simulink model "ObjectTrackerHDL_ew"  (R2024b)
settings: Solver=VariableStepAuto  StartTime=0.0  StopTime=0.2  RelTol=1e-3  EnableMultiTasking=on
PreLoadFcn:
  | % Blank input
  | img = zeros(480,640);
  | 
  | % Initialize ROI and its center
  | ROI = [175 270 127 127];
  | center = [ROI(2)+(ROI(4)+1)/2 ROI(1)+(ROI(3)+1)/2];
  | 
  | % Template Size
  | templateSize = 128;
  | tSize = templateSize;
  | 
  | % Learning rate
  | eta = 0.075;
  | 
  | % Number of training images
  | trainCount = 2;
  | 
  | % Gaussian Variance
  | sig = 2;
  | 
  | % Generate a Gaussian centered on the first frame
  | iSize = size(img);
  | [x,y] = ndgrid(1:iSize(1), 1:iSize(2));
  | gauss = exp(-((x-center(1)).^2 + (y-center(2)).^2)./(2*sig));
  | gauss = mat2gray(gauss);
  | 
  | % Generate the first template
  | img = imcrop(img, ROI);
  | gauss = imcrop(gauss, ROI);
  | 
  | % Generate the preprocess windowing function
  | [w1,w2] = meshgrid(window(@hann,tSize),window(@hann,tSize));
  | win = w1.*w2;
  | 
  | % Blank initial coefficients
  | G = zeros(tSize,tSize);
  | Ai = zeros(tSize,tSize);
  | Bi = zeros(tSize,tSize);
  | Hi = zeros(tSize,tSize);
  | 
  | numRows = tSize;
  | numCols = tSize;
InitFcn:
  | % Read the first frame
  | vidFReader = VideoReader(get_param('ObjectTrackerHDL/Input','inputFilename'));
  | img = read(vidFReader,1);
  | if (size(img,3) == 3)
  |     img = rgb2gray(img);
  | end
  | img = double(img);
  | 
  | % Initialize Object Center
  | objectCenter = str2num(get_param('ObjectTrackerHDL/ObjectTrackerHDL','objectCenter'));
  | 
  | % Template Size
  | templateSize = str2num(get_param('ObjectTrackerHDL/ObjectTrackerHDL','templateSize'));
  | originROI = objectCenter-templateSize/2;
  | tSize = templateSize;
  | 
  | % Initialize ROI and its center
  | ROI = [originROI tSize-1 tSize-1];
  | center = [ROI(2)+(ROI(4)+1)/2 ROI(1)+(ROI(3)+1)/2];
  | 
  | % Learning rate
  | eta = 0.075;
  | 
  | % Number of training images
  | trainCount = 128;
  | 
  | % Gaussian Variance
  | sig = 2;
  | 
  | % Generate a Gaussian centered on the first frame
  | iSize = size(img);
  | [x,y] = ndgrid(1:iSize(1), 1:iSize(2));
  | gauss = exp(-((x-center(1)).^2 + (y-center(2)).^2)./(2*sig));
  | gauss = mat2gray(gauss);
  | 
  | % Generate the first template
  | img = imcrop(img, ROI);
  | gauss = imcrop(gauss, ROI);
  | 
  | % Generate the preprocess windowing function
  | [w1,w2] = meshgrid(window(@hann,tSize),window(@hann,tSize));
  | win = w1.*w2;
  | 
  | % Preprocessing the first template
  | hgamma = vision.GammaCorrector(2.0,'Correction','De-gamma');
  | img = hgamma(uint8(img));
  | img = double(img);
  | mean1 = mean(img(:));
  | std1 = std(img(:));
  | img = (img-mean1)/std1;
  | fii = img.*win;
  | 
  | % Convert to frequency domain and calculate initial coefficients
  | G = fft2(gauss);
  | Ai = (G.*conj(fft2(fii)));
  | Bi = real((fft2(fii).*conj(fft2(fii))));
  | 
  | rng('default');
  | % Initial training procedure
  | for i = 1:trainCount
  | ... (+19 lines)
model workspace (MAT data in the model file):
  mwTaskManagerKernelLatency = 0
undefined symbols (not defined in the file): a, b, c, Rec, SDTV
libraries: hdlsllib x61, simulink x17, visionhdlutilities x8, visionstatistics x6, dsphdlxfrm2 x6, visionconversions x4, visiontransforms x3, visionhdlio x2, visionhdlconversions x2, visionhdlstatistics x2, visionanalysis x2, visionsinks x1
(part 3 of 3)

== system ObjectTrackerHDL_ew/ObjectTrackerHDL/Track/2-DCorrelation/Prev2-DFFT/pixelBusGenerator ==
  validIn : Inport
  Horizontal : hdlsllib/Sources/HDL Counter  CountType=Count limited  CountInit=0  CountStep=1  CountMax=hEnd  CountFromType=Initial value  CountFrom=0  CountResetPort=off  CountLoadPort=off  CountEnbPort=on  CountDirPort=off  CountHitOutputPort=off  CountDataType=Unsigned  CountWordLen=ceil(log2(hEnd))  CountFracLen=0  CountSampTime=1
  Logical Operator{3..6} (4 alike) : Logic  AllPortsSameDT=off  OutDataTypeStr=boolean
  Pixel Control Bus Creator : visionhdlutilities/Pixel Control Bus Creator
  Vertical : hdlsllib/Sources/HDL Counter  CountType=Count limited  CountInit=0  CountStep=1  CountMax=vEnd  CountFromType=Initial value  CountFrom=0  CountResetPort=off  CountLoadPort=off  CountEnbPort=on  CountDirPort=off  CountHitOutputPort=off  CountDataType=Unsigned  CountWordLen=ceil(log2(vEnd))  CountFracLen=0  CountSampTime=1
  hEnd : simulink/Logic and Bit Operations/Compare To Constant  relop===  const=hEnd  OutDataTypeStr=boolean
  hStart : simulink/Logic and Bit Operations/Compare To Constant  relop===  const=0  OutDataTypeStr=boolean
  vEnd : simulink/Logic and Bit Operations/Compare To Constant  relop===  const=vEnd  OutDataTypeStr=boolean
  vStart : simulink/Logic and Bit Operations/Compare To Constant  relop===  const=0  OutDataTypeStr=boolean
  busOut : Outport  VectorParamsAs1DForOutWhenUnconnected=off
  frameDone : Outport  Port=2  VectorParamsAs1DForOutWhenUnconnected=off
  wires:
  validIn/1 -> Pixel Control Bus Creator/5, Vertical/1, Logical Operator4/1, Logical Operator5/1, Logical Operator6/1, Logical Operator3/1, Horizontal/1
  Horizontal/1 -> hEnd/1, hStart/1
  hEnd/1 -> Logical Operator4/2
  Vertical/1 -> vStart/1, vEnd/1
  vStart/1 -> Logical Operator5/2
  vEnd/1 -> Logical Operator6/2
  Logical Operator5/1 -> Pixel Control Bus Creator/3
  Logical Operator3/1 -> Pixel Control Bus Creator/1
  Logical Operator4/1 -> Pixel Control Bus Creator/2
  hStart/1 -> Logical Operator3/2
  Logical Operator6/1 -> frameDone/1, Pixel Control Bus Creator/4
  Pixel Control Bus Creator/1 -> busOut/1

== system ObjectTrackerHDL_ew/ObjectTrackerHDL/Track/2-DCorrelation/2-DIFFT/CornerTurnMemory/BankBit ==
  addrIn : Inport
  Bit Slice1 : hdlsllib/Logic and Bit Operations/Bit Slice  lidx=(log2(numCols)+log2(numRows))  ridx=(log2(numCols)+log2(numRows))
  Logical Operator3 : Logic  Operator=NOT  IconShape=distinctive  AllPortsSameDT=off  OutDataTypeStr=boolean
  bankWr : Outport  VectorParamsAs1DForOutWhenUnconnected=off
  wires:
  Logical Operator3/1 -> bankWr/1
  Bit Slice1/1 -> Logical Operator3/1
  addrIn/1 -> Bit Slice1/1

== system ObjectTrackerHDL_ew/ObjectTrackerHDL/Track/2-DCorrelation/2-DIFFT/CornerTurnMemory/LowerRAM ==
  din : Inport
  wr_addr : Inport  Port=2
  wr_en : Inport  Port=3
  rd_addr : Inport  Port=4
  complexDataConcat : MATLABSystem  System=hdl.RAM  RAMType=Simple dual port  AsyncRead=off  WriteOutputValue=New data  RAMInitialValue=0  allowBusInputs=off  WritesHaveOutput=on  NumReads=0  NumWrites=1  SimulateUsing=Code generation  ModelRAMDelay=on
      mask Type: hdl.RAM
      mask Display:
      | disp(['Simple' char(10) 'Dual Port' char(10) 'RAM']);
      | port_label('input',1,'din');
      | port_label('input',2,'wr_addr');
      | port_label('input',3,'we');
      | port_label('input',4,'rd_addr');
      | port_label('output',1,'dout');
  dout : Outport  VectorParamsAs1DForOutWhenUnconnected=off
  wires:
  wr_addr/1 -> complexDataConcat/2
  wr_en/1 -> complexDataConcat/3
  rd_addr/1 -> complexDataConcat/4
  din/1 -> complexDataConcat/1
  complexDataConcat/1 -> dout/1

== system ObjectTrackerHDL_ew/ObjectTrackerHDL/Track/2-DCorrelation/2-DIFFT/CornerTurnMemory/SwapAddr ==
  addrIn : Inport
  Bit Concat : hdlsllib/Logic and Bit Operations/Bit Concat  numInputs=2
  Bit Shift : hdlsllib/Logic and Bit Operations/Bit Shift  mode=Shift Left Logical  N=log2(numCols)
  Bit Slice : hdlsllib/Logic and Bit Operations/Bit Slice  lidx=(log2(numCols)+log2(numRows))-1  ridx=log2(numCols)
  Logical Operator3 : Logic  Operator=NOT  IconShape=distinctive  AllPortsSameDT=off  OutDataTypeStr=boolean
  bankBit : hdlsllib/Logic and Bit Operations/Bit Slice  lidx=(log2(numCols)+log2(numRows))  ridx=(log2(numCols)+log2(numRows))
  upperBits : hdlsllib/Logic and Bit Operations/Bit Slice  lidx=(log2(numCols)+log2(numRows))-1  ridx=log2(numCols)
  bankRd : Outport  VectorParamsAs1DForOutWhenUnconnected=off
  addrRd : Outport  Port=2  VectorParamsAs1DForOutWhenUnconnected=off
  wires:
  Bit Concat/1 -> addrRd/1
  upperBits/1 -> Bit Concat/2
  addrIn/1 -> Bit Shift/1, bankBit/1, upperBits/1
  bankBit/1 -> Logical Operator3/1
  Logical Operator3/1 -> bankRd/1
  Bit Shift/1 -> Bit Slice/1
  Bit Slice/1 -> Bit Concat/1

== system ObjectTrackerHDL_ew/ObjectTrackerHDL/Track/2-DCorrelation/2-DIFFT/CornerTurnMemory/UpperRAM ==
  din : Inport
  wr_addr : Inport  Port=2
  wr_en : Inport  Port=3
  rd_addr : Inport  Port=4
  complexDataConcat : MATLABSystem  System=hdl.RAM  RAMType=Simple dual port  AsyncRead=off  WriteOutputValue=New data  RAMInitialValue=0  allowBusInputs=off  WritesHaveOutput=on  NumReads=0  NumWrites=1  SimulateUsing=Code generation  ModelRAMDelay=on
      mask Type: hdl.RAM
      mask Display:
      | disp(['Simple' char(10) 'Dual Port' char(10) 'RAM']);
      | port_label('input',1,'din');
      | port_label('input',2,'wr_addr');
      | port_label('input',3,'we');
      | port_label('input',4,'rd_addr');
      | port_label('output',1,'dout');
  dout : Outport  VectorParamsAs1DForOutWhenUnconnected=off
  wires:
  complexDataConcat/1 -> dout/1
  din/1 -> complexDataConcat/1
  rd_addr/1 -> complexDataConcat/4
  wr_en/1 -> complexDataConcat/3
  wr_addr/1 -> complexDataConcat/2

== system ObjectTrackerHDL_ew/ObjectTrackerHDL/Track/2-DCorrelation/CoefficientsUpdate/CoefficientsUpdate/ComplexDivide ==
  Dividend : Inport
  Divisor : Inport  Port=2
  Complex to Real-Imag : ComplexToRealImag
  Data Type Conversion : DataTypeConversion  OutDataTypeStr=fixdt(1,44,16)  SaturateOnIntegerOverflow=off  RndMeth=Floor
  Data Type Conversion1 : DataTypeConversion  OutDataTypeStr=fixdt(1,44,16)  SaturateOnIntegerOverflow=off  RndMeth=Floor
  Delay14 : Delay  DelayLength=1+52  InitialCondition=0
  Delay15 : Delay  DelayLength=1+52  InitialCondition=0
  Divide3 : Product  Inputs=*/  OutDataTypeStr=fixdt(1,24,12)  RndMeth=Simplest  SaturateOnIntegerOverflow=on
  Divide4 : Product  Inputs=*/  OutDataTypeStr=fixdt(1,24,12)  RndMeth=Simplest  SaturateOnIntegerOverflow=on
  Real-Imag to Complex : RealImagToComplex
  Quotient : Outport
  wires:
  Divide3/1 -> Delay14/1
  Dividend/1 -> Complex to Real-Imag/1
  Data Type Conversion1/1 -> Divide4/1
  Complex to Real-Imag/2 -> Data Type Conversion1/1
  Delay14/1 -> Real-Imag to Complex/1
  Real-Imag to Complex/1 -> Quotient/1
  Data Type Conversion/1 -> Divide3/1
  Delay15/1 -> Real-Imag to Complex/2
  Divisor/1 -> Divide4/2, Divide3/2
  Divide4/1 -> Delay15/1
  Complex to Real-Imag/1 -> Data Type Conversion/1

== system ObjectTrackerHDL_ew/ObjectTrackerHDL/Track/2-DCorrelation/Curr2-DFFT/CornerTurnMemory/BankBit ==
  addrIn : Inport
  Bit Slice1 : hdlsllib/Logic and Bit Operations/Bit Slice  lidx=(log2(numCols)+log2(numRows))  ridx=(log2(numCols)+log2(numRows))
  Logical Operator3 : Logic  Operator=NOT  IconShape=distinctive  AllPortsSameDT=off  OutDataTypeStr=boolean
  bankWr : Outport  VectorParamsAs1DForOutWhenUnconnected=off
  wires:
  Logical Operator3/1 -> bankWr/1
  Bit Slice1/1 -> Logical Operator3/1
  addrIn/1 -> Bit Slice1/1

== system ObjectTrackerHDL_ew/ObjectTrackerHDL/Track/2-DCorrelation/Curr2-DFFT/CornerTurnMemory/LowerRAM ==
  din : Inport
  wr_addr : Inport  Port=2
  wr_en : Inport  Port=3
  rd_addr : Inport  Port=4
  complexDataConcat : MATLABSystem  System=hdl.RAM  RAMType=Simple dual port  AsyncRead=off  WriteOutputValue=New data  RAMInitialValue=0  allowBusInputs=off  WritesHaveOutput=on  NumReads=0  NumWrites=1  SimulateUsing=Code generation  ModelRAMDelay=on
      mask Type: hdl.RAM
      mask Display:
      | disp(['Simple' char(10) 'Dual Port' char(10) 'RAM']);
      | port_label('input',1,'din');
      | port_label('input',2,'wr_addr');
      | port_label('input',3,'we');
      | port_label('input',4,'rd_addr');
      | port_label('output',1,'dout');
  dout : Outport  VectorParamsAs1DForOutWhenUnconnected=off
  wires:
  wr_addr/1 -> complexDataConcat/2
  wr_en/1 -> complexDataConcat/3
  rd_addr/1 -> complexDataConcat/4
  din/1 -> complexDataConcat/1
  complexDataConcat/1 -> dout/1

== system ObjectTrackerHDL_ew/ObjectTrackerHDL/Track/2-DCorrelation/Curr2-DFFT/CornerTurnMemory/SwapAddr ==
  addrIn : Inport
  Bit Concat : hdlsllib/Logic and Bit Operations/Bit Concat  numInputs=2
  Bit Shift : hdlsllib/Logic and Bit Operations/Bit Shift  mode=Shift Left Logical  N=log2(numCols)
  Bit Slice : hdlsllib/Logic and Bit Operations/Bit Slice  lidx=(log2(numCols)+log2(numRows))-1  ridx=log2(numCols)
  Logical Operator3 : Logic  Operator=NOT  IconShape=distinctive  AllPortsSameDT=off  OutDataTypeStr=boolean
  bankBit : hdlsllib/Logic and Bit Operations/Bit Slice  lidx=(log2(numCols)+log2(numRows))  ridx=(log2(numCols)+log2(numRows))
  upperBits : hdlsllib/Logic and Bit Operations/Bit Slice  lidx=(log2(numCols)+log2(numRows))-1  ridx=log2(numCols)
  bankRd : Outport  VectorParamsAs1DForOutWhenUnconnected=off
  addrRd : Outport  Port=2  VectorParamsAs1DForOutWhenUnconnected=off
  wires:
  Bit Concat/1 -> addrRd/1
  upperBits/1 -> Bit Concat/2
  addrIn/1 -> Bit Shift/1, bankBit/1, upperBits/1
  bankBit/1 -> Logical Operator3/1
  Logical Operator3/1 -> bankRd/1
  Bit Shift/1 -> Bit Slice/1
  Bit Slice/1 -> Bit Concat/1

== system ObjectTrackerHDL_ew/ObjectTrackerHDL/Track/2-DCorrelation/Curr2-DFFT/CornerTurnMemory/UpperRAM ==
  din : Inport
  wr_addr : Inport  Port=2
  wr_en : Inport  Port=3
  rd_addr : Inport  Port=4
  complexDataConcat : MATLABSystem  System=hdl.RAM  RAMType=Simple dual port  AsyncRead=off  WriteOutputValue=New data  RAMInitialValue=0  allowBusInputs=off  WritesHaveOutput=on  NumReads=0  NumWrites=1  SimulateUsing=Code generation  ModelRAMDelay=on
      mask Type: hdl.RAM
      mask Display:
      | disp(['Simple' char(10) 'Dual Port' char(10) 'RAM']);
      | port_label('input',1,'din');
      | port_label('input',2,'wr_addr');
      | port_label('input',3,'we');
      | port_label('input',4,'rd_addr');
      | port_label('output',1,'dout');
  dout : Outport  VectorParamsAs1DForOutWhenUnconnected=off
  wires:
  complexDataConcat/1 -> dout/1
  din/1 -> complexDataConcat/1
  rd_addr/1 -> complexDataConcat/4
  wr_en/1 -> complexDataConcat/3
  wr_addr/1 -> complexDataConcat/2

== system ObjectTrackerHDL_ew/ObjectTrackerHDL/Track/2-DCorrelation/Prev2-DFFT/CornerTurnMemory/BankBit ==
  addrIn : Inport
  Bit Slice1 : hdlsllib/Logic and Bit Operations/Bit Slice  lidx=(log2(numCols)+log2(numRows))  ridx=(log2(numCols)+log2(numRows))
  Logical Operator3 : Logic  Operator=NOT  IconShape=distinctive  AllPortsSameDT=off  OutDataTypeStr=boolean
  bankWr : Outport  VectorParamsAs1DForOutWhenUnconnected=off
  wires:
  Logical Operator3/1 -> bankWr/1
  Bit Slice1/1 -> Logical Operator3/1
  addrIn/1 -> Bit Slice1/1

== system ObjectTrackerHDL_ew/ObjectTrackerHDL/Track/2-DCorrelation/Prev2-DFFT/CornerTurnMemory/LowerRAM ==
  din : Inport
  wr_addr : Inport  Port=2
  wr_en : Inport  Port=3
  rd_addr : Inport  Port=4
  complexDataConcat : MATLABSystem  System=hdl.RAM  RAMType=Simple dual port  AsyncRead=off  WriteOutputValue=New data  RAMInitialValue=0  allowBusInputs=off  WritesHaveOutput=on  NumReads=0  NumWrites=1  SimulateUsing=Code generation  ModelRAMDelay=on
      mask Type: hdl.RAM
      mask Display:
      | disp(['Simple' char(10) 'Dual Port' char(10) 'RAM']);
      | port_label('input',1,'din');
      | port_label('input',2,'wr_addr');
      | port_label('input',3,'we');
      | port_label('input',4,'rd_addr');
      | port_label('output',1,'dout');
  dout : Outport  VectorParamsAs1DForOutWhenUnconnected=off
  wires:
  wr_addr/1 -> complexDataConcat/2
  wr_en/1 -> complexDataConcat/3
  rd_addr/1 -> complexDataConcat/4
  din/1 -> complexDataConcat/1
  complexDataConcat/1 -> dout/1

== system ObjectTrackerHDL_ew/ObjectTrackerHDL/Track/2-DCorrelation/Prev2-DFFT/CornerTurnMemory/SwapAddr ==
  addrIn : Inport
  Bit Concat : hdlsllib/Logic and Bit Operations/Bit Concat  numInputs=2
  Bit Shift : hdlsllib/Logic and Bit Operations/Bit Shift  mode=Shift Left Logical  N=log2(numCols)
  Bit Slice : hdlsllib/Logic and Bit Operations/Bit Slice  lidx=(log2(numCols)+log2(numRows))-1  ridx=log2(numCols)
  Logical Operator3 : Logic  Operator=NOT  IconShape=distinctive  AllPortsSameDT=off  OutDataTypeStr=boolean
  bankBit : hdlsllib/Logic and Bit Operations/Bit Slice  lidx=(log2(numCols)+log2(numRows))  ridx=(log2(numCols)+log2(numRows))
  upperBits : hdlsllib/Logic and Bit Operations/Bit Slice  lidx=(log2(numCols)+log2(numRows))-1  ridx=log2(numCols)
  bankRd : Outport  VectorParamsAs1DForOutWhenUnconnected=off
  addrRd : Outport  Port=2  VectorParamsAs1DForOutWhenUnconnected=off
  wires:
  Bit Concat/1 -> addrRd/1
  upperBits/1 -> Bit Concat/2
  addrIn/1 -> Bit Shift/1, bankBit/1, upperBits/1
  bankBit/1 -> Logical Operator3/1
  Logical Operator3/1 -> bankRd/1
  Bit Shift/1 -> Bit Slice/1
  Bit Slice/1 -> Bit Concat/1

== system ObjectTrackerHDL_ew/ObjectTrackerHDL/Track/2-DCorrelation/Prev2-DFFT/CornerTurnMemory/UpperRAM ==
  din : Inport
  wr_addr : Inport  Port=2
  wr_en : Inport  Port=3
  rd_addr : Inport  Port=4
  complexDataConcat : MATLABSystem  System=hdl.RAM  RAMType=Simple dual port  AsyncRead=off  WriteOutputValue=New data  RAMInitialValue=0  allowBusInputs=off  WritesHaveOutput=on  NumReads=0  NumWrites=1  SimulateUsing=Code generation  ModelRAMDelay=on
      mask Type: hdl.RAM
      mask Display:
      | disp(['Simple' char(10) 'Dual Port' char(10) 'RAM']);
      | port_label('input',1,'din');
      | port_label('input',2,'wr_addr');
      | port_label('input',3,'we');
      | port_label('input',4,'rd_addr');
      | port_label('output',1,'dout');
  dout : Outport  VectorParamsAs1DForOutWhenUnconnected=off
  wires:
  complexDataConcat/1 -> dout/1
  din/1 -> complexDataConcat/1
  rd_addr/1 -> complexDataConcat/4
  wr_en/1 -> complexDataConcat/3
  wr_addr/1 -> complexDataConcat/2

== matlab function ObjectTrackerHDL_ew/ObjectTrackerHDL/Track/2-DCorrelation/Prev2-DFFT/CornerTurnMemory/CounterDelay ==
  settings: fimath=hdlfimath
  data: vld_in input boolean; vld_out output boolean; DELAY parameter; templateSize parameter; blanking parameter
function vld_out = cntr_delay(vld_in, DELAY, templateSize, blanking)

CNTR_NT = numerictype(0,nextpow2(DELAY+2),0);
FCNTR_NT = numerictype(0,nextpow2(DELAY),0);
FM = hdlfimath;

persistent wr_cntr rd_cntr rdrw_cntr rdbl_cntr flush_cntr state

STATE_FILL = coder.const(0);
STATE_FLUSH = coder.const(1);
STATE_RESET = coder.const(3);

if isempty(wr_cntr)
    wr_cntr = fi(0,CNTR_NT, FM);
    rd_cntr = fi(0,CNTR_NT, FM);
    rdrw_cntr = fi(0,CNTR_NT, FM);
    rdbl_cntr = fi(0,CNTR_NT, FM);
    flush_cntr = fi(0,FCNTR_NT,FM);
    state = fi(STATE_FILL, 0, 2, 0);
end

%dcount = fi(wr_cntr-rd_cntr,CNTR_NT, FM);

vld_out = false;

switch state
    case STATE_FILL
        if wr_cntr == DELAY
            vld_out = true;
            state(:) = STATE_FLUSH;
            flush_cntr(:) = DELAY-1;
            rd_cntr(:) = rd_cntr + 1;
            rdrw_cntr(:) = rdrw_cntr + 1;
            wr_cntr(:) = 0;
        else
            vld_out = false;
        end
    case STATE_FLUSH
        if flush_cntr == 1
            state(:) = STATE_RESET;
        end 
        if rdrw_cntr < templateSize
        rd_cntr(:) = rd_cntr + 1;
        rdrw_cntr(:) = rdrw_cntr + 1;
        flush_cntr(:) = flush_cntr -1;
        vld_out = true;
        else
        rdbl_cntr(:) = rdbl_cntr(:) + 1;
        vld_out = false;
        end
        if rdbl_cntr >=(blanking-templateSize)
        rdrw_cntr(:) = 0;
        rdbl_cntr(:) = 0;
        end
    case STATE_RESET
        if wr_cntr == DELAY %* 2 -1 
            state(:) = STATE_FILL;
%          if rd_cntr ~= DELAY
%              disp(rd_cntr);
%             error('Out of sync Counter (RD)');
%          end
         rd_cntr(:) = 0;
%          if wr_cntr ~= DELAY
%              disp(wr_cntr);
%             error('Out of sync Counter (WR)');
%          end
        %wr_cntr(:) = 0;
        flush_cntr(:) = DELAY-1;
        else 
            state(:) = STATE_RESET;
        end
end

if vld_in
    wr_cntr(:) = wr_cntr + 1;
end

== matlab function ObjectTrackerHDL_ew/ObjectTrackerHDL/Overlay/VideoOverlay/MATLAB Function ==
  data: position input; Color output; AddShape output; rowCount input; colCount input; colorValue input; lineWidth input
function [Color, AddShape] = InsertRectangle(position, rowCount, colCount, colorValue, lineWidth)
%#codegen


halfLineWidth = int32(bitshift(lineWidth,-1));

Color = uint8(colorValue);%[255 255 0]
% position must not be a column vector
% [x y width]
objectLocAndWidth = int32(position(:,1:4));
objectLocTopStart = objectLocAndWidth(:,1) - int32(halfLineWidth);
objectLocTopEnd = objectLocAndWidth(:,1) + int32(halfLineWidth);
objectLocBottomStart = objectLocAndWidth(:,1) - int32(halfLineWidth)+ objectLocAndWidth(:,3);
objectLocBottomEnd = objectLocAndWidth(:,1) + int32(halfLineWidth)+ objectLocAndWidth(:,3);
objectLocLeftStart = objectLocAndWidth(:,2) - int32(halfLineWidth);
objectLocLeftEnd = objectLocAndWidth(:,2) + int32(halfLineWidth);
objectLocRightStart = objectLocAndWidth(:,2) - int32(halfLineWidth) + objectLocAndWidth(:,4);
objectLocRightEnd = objectLocAndWidth(:,2) + int32(halfLineWidth) + objectLocAndWidth(:,4);

AddShapeHorLimit = (rowCount>=objectLocTopStart) & (rowCount<=objectLocBottomEnd);
AddShapeVerLimit = (colCount>=objectLocLeftStart) & (colCount<=objectLocRightEnd);

AddShapeHor = ((((rowCount>=objectLocTopStart) & (rowCount<=objectLocTopEnd)) | ((rowCount>=objectLocBottomStart) & (rowCount<=objectLocBottomEnd))) & AddShapeVerLimit);
AddShapeVer = ((((colCount>=objectLocLeftStart) & (colCount<=objectLocLeftEnd)) | ((colCount>=objectLocRightStart) & (colCount<=objectLocRightEnd))) & AddShapeHorLimit);
AddShape = AddShapeHor | AddShapeVer;

end


% for(int x=0; x < bufferedImage.getWidth(); x++) {
%             for(int y=0; y < bufferedImage.getHeight(); y++) {
%                 R1 = BufferedImageGetPixelARGB(bufferedImage, "R", x, y);
%                 G1 = BufferedImageGetPixelARGB(bufferedImage, "G", x, y);
%                 B1 = BufferedImageGetPixelARGB(bufferedImage, "B", x, y);
%                 W1 = Math.min(R1, Math.min(G1, B1));
%                 W2 = Math.min(R2, Math.min(G2, B2));
%                 R1 -= W1;
%                 G1 -= W1;
%                 B1 -= W1;
%                 R2 -= W2;
%                 G2 -= W2;
%                 M1 = Math.max(R1, Math.max(G1, B1));
%                 M2 = Math.max(R2, Math.max(G2, B2));
%                 br = (M1 + M2)/(2*BufferedImageGetPixelARGB(bufferedImage, "A", x, y));
%                 R3 = (int) ((R1 + R2) * br);
%                 G3 = (int) ((G1 + G2) * br);
%                 B3 = (int) ((B1 + B2) * br);
%                 W3 = (W1 + W2) / 2;
%                 R3 += W3;
%                 G3 += W3;
%                 B3 += W3;
%                 newImage.setRGB(x, y, RGBValuesToInt(R3, G3, B3));
%             }
%         }

== matlab function ObjectTrackerHDL_ew/ObjectTrackerHDL/Track/2-DCorrelation/Curr2-DFFT/CornerTurnMemory/CounterDelay ==
  settings: fimath=hdlfimath
  data: vld_in input boolean; vld_out output boolean; DELAY parameter; templateSize parameter; blanking parameter
function vld_out = cntr_delay(vld_in, DELAY, templateSize, blanking)

CNTR_NT = numerictype(0,nextpow2(DELAY+2),0);
FCNTR_NT = numerictype(0,nextpow2(DELAY),0);
FM = hdlfimath;

persistent wr_cntr rd_cntr rdrw_cntr rdbl_cntr flush_cntr state

STATE_FILL = coder.const(0);
STATE_FLUSH = coder.const(1);
STATE_RESET = coder.const(3);

if isempty(wr_cntr)
    wr_cntr = fi(0,CNTR_NT, FM);
    rd_cntr = fi(0,CNTR_NT, FM);
    rdrw_cntr = fi(0,CNTR_NT, FM);
    rdbl_cntr = fi(0,CNTR_NT, FM);
    flush_cntr = fi(0,FCNTR_NT,FM);
    state = fi(STATE_FILL, 0, 2, 0);
end

%dcount = fi(wr_cntr-rd_cntr,CNTR_NT, FM);

vld_out = false;

switch state
    case STATE_FILL
        if wr_cntr == DELAY
            vld_out = true;
            state(:) = STATE_FLUSH;
            flush_cntr(:) = DELAY-1;
            rd_cntr(:) = rd_cntr + 1;
            rdrw_cntr(:) = rdrw_cntr + 1;
            wr_cntr(:) = 0;
        else
            vld_out = false;
        end
    case STATE_FLUSH
        if flush_cntr == 1
            state(:) = STATE_RESET;
        end 
        if rdrw_cntr < templateSize
        rd_cntr(:) = rd_cntr + 1;
        rdrw_cntr(:) = rdrw_cntr + 1;
        flush_cntr(:) = flush_cntr -1;
        vld_out = true;
        else
        rdbl_cntr(:) = rdbl_cntr(:) + 1;
        vld_out = false;
        end
        if rdbl_cntr >=(blanking-templateSize)
        rdrw_cntr(:) = 0;
        rdbl_cntr(:) = 0;
        end
    case STATE_RESET
        if wr_cntr == DELAY %* 2 -1 
            state(:) = STATE_FILL;
%          if rd_cntr ~= DELAY
%              disp(rd_cntr);
%             error('Out of sync Counter (RD)');
%          end
         rd_cntr(:) = 0;
%          if wr_cntr ~= DELAY
%              disp(wr_cntr);
%             error('Out of sync Counter (WR)');
%          end
        %wr_cntr(:) = 0;
        flush_cntr(:) = DELAY-1;
        else 
            state(:) = STATE_RESET;
        end
end

if vld_in
    wr_cntr(:) = wr_cntr + 1;
end

== matlab function ObjectTrackerHDL_ew/Display/VideoOverlay ==
  data: img input; y output; ROI input
function y = fcn(img, ROI)
img = insertShape(img, 'Rectangle', ROI, 'LineWidth', 2);
img =insertText(img, [1 1],'Behavioral','FontSize',15,'BoxColor',...
        [255 255 0],'BoxOpacity',0.7,'TextColor',[255 255 255]);
img =insertText(img, [1 30],'HDL','FontSize',15,'BoxColor',...
        [0 0 255],'BoxOpacity',0.7,'TextColor',[255 255 255]);
y = img;

== matlab function ObjectTrackerHDL_ew/Behavioral/Preprocess/MATLAB Function1 ==
  data: img input; fi output size=[templateSize templateSize]; ROI input; templateSize parameter
function fi = crop(img, ROI, templateSize)
fi = uint8(zeros(templateSize));
coder.extrinsic('imcrop');
fi = imcrop(img, ROI);

== matlab function ObjectTrackerHDL_ew/Subsystem/MATLAB Function ==
  data: inputImage input; outputImage output
function outputImage = applyCLAHE(inputImage)
% Input: inputImage - Grayscale image
% Output: outputImage - Image after CLAHE

    % Apply CLAHE using MATLAB's built-in function
    % Ensure inputImage is in the range [0, 1]
    inputImage = mat2gray(inputImage); 
    outputImage = adapthisteq(inputImage, 'ClipLimit', 0.01, 'NumTiles', [8 8]);
end

== matlab function ObjectTrackerHDL_ew/Subsystem/MATLAB Function1 ==
  data: edgeImage input; objectCenter output; templateSize output; edgeImage output
function [objectCenter, templateSize,edgeImage] = calculateROI(edgeImage)
%#codegen

    % Output dimensions and default values
    objectCenter = zeros(1, 2, 'double');  % [1x2] row vector
    templateSize = 128;                   % Default scalar size

    % Ensure edgeImage is logical for regionprops compatibility
    edgeImage = logical(edgeImage);

    % Perform morphological filtering to remove noise
    se = strel('disk', 5);                % Structuring element for morphological operations
    edgeImage = imopen(edgeImage, se);    % Open operation to remove noise
    edgeImage = imclose(edgeImage, se);   % Close operation to fill gaps

    % Save intermediate edgeImage to workspace for debugging
    %assignin('base', 'edgeImage_morphed', edgeImage);

    % Fill holes and remove small objects
    edgeImage = imfill(edgeImage, 'holes'); % Fill interior gaps
    edgeImage = bwareaopen(edgeImage, 1000); % Remove small objects with area < 1000

    % Save final processed edgeImage to workspace for debugging
    assignin('base', 'edgeImage_processed', edgeImage);

    % Perform blob analysis on the filtered binary image
    stats = regionprops(edgeImage, 'Centroid', 'BoundingBox', 'Area');

    % Ensure compatibility with MATLAB Coder
    coder.varsize('stats', [100, 1]);     % Limit to a maximum of 100 objects

    % Minimum area threshold to filter out small/noisy blobs
    minArea = 500; % Adjusted for larger objects like airplanes
    validStats = stats([stats.Area] > minArea);

    % Check if valid objects exist
    if ~isempty(validStats)
        % Extract Area values
        areaValues = [validStats.Area];

        % Select the largest detected object
        [~, idx] = max(areaValues);       % Select the index of the largest area

        centroid = validStats(idx).Centroid;    % [x, y] center of the largest blob
        bbox = validStats(idx).BoundingBox;     % Bounding box of the blob

        % Assign outputs
        objectCenter(1) = centroid(1);          % x-coordinate of the center
        objectCenter(2) = centroid(2);          % y-coordinate of the center

        % Calculate templateSize and snap to nearest valid value
        maxDimension = max(bbox(3:4));          % Use largest dimension of bounding box
        validSizes = [16, 32, 64, 128, 256];    % Allowed sizes
        [~, idx] = min(abs(validSizes - maxDimension)); % Find closest valid size
        templateSize = validSizes(idx);         % Snap to nearest valid size
    end

    % Visualization for debugging
    if coder.target('MATLAB') % Only works during MATLAB simulation
        figure;
        imshow(edgeImage);
        hold on;
        if exist('bbox', 'var')
            rectangle('Position', bbox, 'EdgeColor', 'r', 'LineWidth', 2);
            plot(objectCenter(1), objectCenter(2), 'b*', 'MarkerSize', 10);
        end
        hold off;
        title('Detected Object and ROI');
    end
end

== matlab function ObjectTrackerHDL_ew/Behavioral/Preprocess/MATLAB Function7 ==
  data: img input; fi output size=[templateSize templateSize]; ROI input; templateSize parameter
function fi = crop(img, ROI, templateSize)
fi = uint8(zeros(templateSize));
coder.extrinsic('imcrop');
fi = imcrop(img, ROI);

== matlab function ObjectTrackerHDL_ew/ObjectTrackerHDL/Track/2-DCorrelation/2-DIFFT/CornerTurnMemory/CounterDelay ==
  settings: fimath=hdlfimath
  data: vld_in input boolean; vld_out output boolean; DELAY parameter; templateSize parameter; blanking parameter
function vld_out = cntr_delay(vld_in, DELAY, templateSize, blanking)

CNTR_NT = numerictype(0,nextpow2(DELAY+2),0);
FCNTR_NT = numerictype(0,nextpow2(DELAY),0);
FM = hdlfimath;

persistent wr_cntr rd_cntr rdrw_cntr rdbl_cntr flush_cntr state

STATE_FILL = coder.const(0);
STATE_FLUSH = coder.const(1);
STATE_RESET = coder.const(3);

if isempty(wr_cntr)
    wr_cntr = fi(0,CNTR_NT, FM);
    rd_cntr = fi(0,CNTR_NT, FM);
    rdrw_cntr = fi(0,CNTR_NT, FM);
    rdbl_cntr = fi(0,CNTR_NT, FM);
    flush_cntr = fi(0,FCNTR_NT,FM);
    state = fi(STATE_FILL, 0, 2, 0);
end

%dcount = fi(wr_cntr-rd_cntr,CNTR_NT, FM);

vld_out = false;

switch state
    case STATE_FILL
        if wr_cntr == DELAY
            vld_out = true;
            state(:) = STATE_FLUSH;
            flush_cntr(:) = DELAY-1;
            rd_cntr(:) = rd_cntr + 1;
            rdrw_cntr(:) = rdrw_cntr + 1;
            wr_cntr(:) = 0;
        else
            vld_out = false;
        end
    case STATE_FLUSH
        if flush_cntr == 1
            state(:) = STATE_RESET;
        end 
        if rdrw_cntr < templateSize
        rd_cntr(:) = rd_cntr + 1;
        rdrw_cntr(:) = rdrw_cntr + 1;
        flush_cntr(:) = flush_cntr -1;
        vld_out = true;
        else
        rdbl_cntr(:) = rdbl_cntr(:) + 1;
        vld_out = false;
        end
        if rdbl_cntr >=(blanking-templateSize)
        rdrw_cntr(:) = 0;
        rdbl_cntr(:) = 0;
        end
    case STATE_RESET
        if wr_cntr == DELAY %* 2 -1 
            state(:) = STATE_FILL;
%          if rd_cntr ~= DELAY
%              disp(rd_cntr);
%             error('Out of sync Counter (RD)');
%          end
         rd_cntr(:) = 0;
%          if wr_cntr ~= DELAY
%              disp(wr_cntr);
%             error('Out of sync Counter (WR)');
%          end
        %wr_cntr(:) = 0;
        flush_cntr(:) = DELAY-1;
        else 
            state(:) = STATE_RESET;
        end
end

if vld_in
    wr_cntr(:) = wr_cntr + 1;
end

== matlab function ObjectTrackerHDL_ew/Behavioral/Track/MaxCorrelation/MATLAB Function13 ==
  data: P output size=[tSize tSize]; gi input size=[tSize tSize]; Q output size=[tSize tSize]
function [P, Q] = findMax(gi)
maxval = max(gi(:));
[P, Q] = find(gi == maxval);
